simulink model "test4"  (R2021a)
settings: Solver=VariableStepAuto  StartTime=0.0  StopTime=20  RelTol=1e-1
undefined symbols (not defined in the file): B_EMB, C1, C_EMB, D_EMB, f, i_EMB, JL, JM, Jm_EMB, K1, N_EMB, rb_EMB, s_EMB, sigbuilder_block, Tc_EMB, Ts_EMB, ub_EMB
libraries: powerlib_extras x9, spsDCVoltageSourceLib x5, spsPermanentMagnetSynchronousMachineLib x5, spsUniversalBridgeLib x5, spspowerguiLib x5, spsVoltageMeasurementLib x4, pid_lib x4, simulink x3, dsparch4 x2, instrumentlib x2, Solver_SF x1
(part 1 of 3)
settings Model: Creator=86188  LastModifiedBy=86188
settings DataIOCC: ReturnWorkspaceOutputs=off

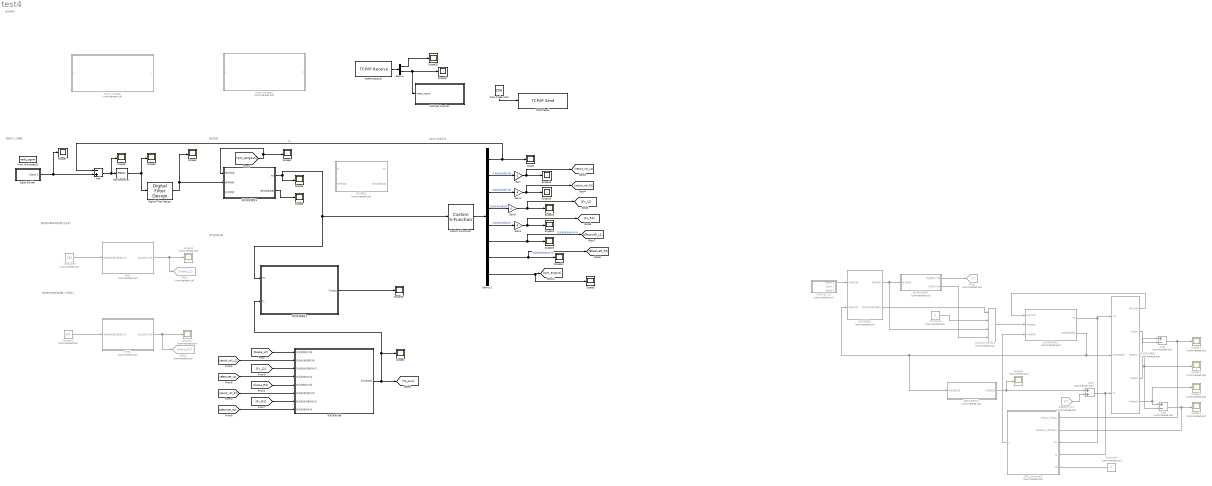
== system test4 ==
  note: 传动系统仿真
  note: 驱动电机
  note: Carsim仿真平台
  note: 驾驶员/工况模型
  note: 线控制动EMB制动器(左后轮)
  note: 线控制动EMB制动器（右后轮）
  note: 驱动电机
  Add : Sum  Inputs=-+
  Add5 : Sum  Commented=on  Inputs=+-
  Add6 : Sum  Commented=on  Inputs=+-
  Add7 : Sum  Commented=on
  CarSim S-Function : Solver_SF/CarSim S-Function  Priority=1  SIMFILE=simfile.sim
  Constant2 : Constant  Commented=on  Value=600
  Constant3 : Constant  Commented=on  Value=0
  Constant4 : Constant  Commented=on  Value=0
  Constant5 : Constant  Commented=on  Value=600
  Demux : Demux  Outputs=2
  Demux1 : Demux  Outputs=8
  Digital Filter Design : dsparch4/Digital Filter Design  mwdsp_browser_bugfix_var=off
  EMB : Subsystem  Commented=on
  EMB1 : Subsystem  Commented=on
  From Workspace1 : FromWorkspace  VariableName=nedc_signal  SampleTime=-1
  Gain{,1,3..4} (4 alike) : Gain  Gain=-1
  Goto : Goto  Commented=on  GotoTag=brake_L2
  Goto1 : Goto  Commented=on  GotoTag=T
  Goto2 : Goto  Commented=on  GotoTag=brake_R2
  MATLAB Function : MATLAB Function  TreatAsAtomicUnit=on
  MPC_controller1 : MATLAB Function  Commented=on  TreatAsAtomicUnit=on
  Multiport Switch1 : MultiPortSwitch  Commented=on  DataPortOrder=Zero-based contiguous  zeroidx=on
  PID Controller : pid_lib/PID Controller  Controller=PID  Form=Parallel  TimeDomain=Continuous-time  UseExternalTs=off  SampleTime=-1  IntegratorMethod=Forward Euler  FilterMethod=Forward Euler  ControllerParametersSource=internal  P=200  I=100  D=0  UseFilter=on  N=100  TunerSelectOption=Transfer Function Based (PID Tuner App)  InitialConditionSource=internal  InitialConditionForIntegrator=0  InitialConditionForFilter=0  DifferentiatorICPrevScaledInput=0  ExternalReset=none  TrackingMode=off  Kt=1  LimitOutput=off  SatLimitsSource=internal  UpperSaturationLimit=3000  LowerSaturationLimit=-3000  LinearizeAsGain=on  AntiWindupMode=none  Kb=1  POutMin=[]  POutMax=[]  IOutMin=[]  IOutMax=[]  DOutMin=[]  DOutMax=[]  NOutMin=[]  NOutMax=[]  SumOutMin=[]  SumOutMax=[]  SaturationOutMin=[]  SaturationOutMax=[]  PParamMin=[]  PParamMax=[]  IParamMin=[]  IParamMax=[]  DParamMin=[]  DParamMax=[]  NParamMin=[]  NParamMax=[]  KbParamMin=[]  KbParamMax=[]  KtParamMin=[]  KtParamMax=[]  KbOutMin=[]  KbOutMax=[]  KtOutMin=[]  KtOutMax=[]  IntegratorOutMin=[]  IntegratorOutMax=[]  FilterOutMin=[]  FilterOutMax=[]  SumI1OutMin=[]  SumI1OutMax=[]  SumI2OutMin=[]  SumI2OutMax=[]  SumI3OutMin=[]  SumI3OutMax=[]  SumI4OutMin=[]  SumI4OutMax=[]  SumDOutMin=[]  SumDOutMax=[]  DifferentiatorOutMin=[]  DifferentiatorOutMax=[]  FilterDiffOutCoefMin=[]  FilterDiffOutCoefMax=[]  ReciprocalOutMin=[]  ReciprocalOutMax=[]  SumDenOutMin=[]  SumDenOutMax=[]  SumNumOutMin=[]  SumNumOutMax=[]  DivideOutMin=[]  DivideOutMax=[]  UdiffTsProdOutMin=[]  UdiffTsProdOutMax=[]  NTsProdOutMin=[]  NTsProdOutMax=[]  UintegralTsProdOutMin=[]  UintegralTsProdOutMax=[]  UngainTsProdOutMin=[]  UngainTsProdOutMax=[]  IntegratorContinuousStateAttributes=''  IntegratorStateMustResolveToSignalObject=off  IntegratorRTWStateStorageClass=Auto  FilterContinuousStateAttributes=''  FilterStateMustResolveToSignalObject=off  FilterRTWStateStorageClass=Auto  ParallelPVariant=InternalParameters  IdealPVariant=Disabled  IVariant=InternalParameters  DVariant=InternalParameters  IntegratorVariant=Continuous  SatVariant=Disabled  AWVariant=Passthrough  PCopyVariant=Disabled  TRVariant=Disabled  FdbkBlocksVariant=Forward  IdealPFdbkVariant=Disabled  SatFdbkVariant=Disabled  DerivativeFilterVariant=ContFilter  NVariant=InternalParameters  NCopyVariant=Disabled  FilterICVariant=InternalICsFilter  IntegratorICVariant=InternalICs  ExternalResetVariant=Disabled  TRSumVariant=Passthrough  SumFdbkVariant=Disabled  SumVariant=Sum_PID  TsampFilterVariant=InternalTs  TsampNgainVariant=Passthrough  TsampIntegralVariant=Passthrough  ExternalSaturationOutDataTypeStr=Inherit: Same as second input
  Scope{,1..9,16..19,21..25} (19 alike) : Scope
  Scope{10..15,20} (7 alike) : Scope  Commented=on
  Signal Builder : Subsystem  Tag=STV Subsys  LoadFcn=sigbuilder_block('load');  StartFcn=sigbuilder_block('start');  StopFcn=sigbuilder_block('stop');  ClipboardFcn=sigbuilder_block('clipboard');  mask(Sigbuilder block){tuvar=[0:10]}
      mask help: Simulink:masks:SigbuilderBlock_MD
      mask init:
      | if ~strcmp(get_param(bdroot(gcbh),'SimulationStatus'),'stopped') tuvar = sigbuilder_block('maskInit'); end
      settings: CopyFcn=sigbuilder_block('copy');  DeleteFcn=sigbuilder_block('delete');  ModelCloseFcn=sigbuilder_block('modelClose');  PreSaveFcn=sigbuilder_block('preSave');  PauseFcn=sigbuilder_block('pause');  ContinueFcn=sigbuilder_block('continue');  NameChangeFcn=sigbuilder_block('namechange');  OpenFcn=sigbuilder_block('open',[86.4 109.2 550.8 400.2 ]);  CloseFcn=sigbuilder_block('close');
      mask Display: plot(0, 0, 100, 100,[2, 2, 32, 32, 2], [68, 8, 8, 68, 68],[32, 2], [38, 38], [32, 19, 2],[53, 60, 44], [32, 17, 17, 2],[16, 16, 31, 31]);txt = getActiveGroup(gcbh);text(2, 100, txt,'verticalAlignment', 'top');
  TCP/IP Receive : instrumentlib/TCP//IP Receive  Host=127.0.0.1  Port=50001  DataSize="[1  2]"  EnableBlockingMode=on  Timeout=10  SampleTime=0.01  DataType=double  ByteOrder=LittleEndian  ASCIIFormatting=%f,  Terminator=LF
  TCP/IP Send : instrumentlib/TCP//IP Send  Host=127.0.0.1  Port=50000  EnableBlockingMode=on  Timeout=10  ByteOrder=LittleEndian  TransferDelay=on
  Zero-Order Hold : ZeroOrderHold  SampleTime=0.01
  brake_strategy : MATLAB Function  Commented=on  TreatAsAtomicUnit=on
  brake_strategy1 : MATLAB Function  Commented=on  TreatAsAtomicUnit=on
  传动系统模型1 : Subsystem
  传动系统模型2 : Subsystem  Commented=on
  复合制动策略1 : Subsystem  Commented=on
  机械制动力矩1 : From  Commented=on  GotoTag=T
  电机模型1 : Subsystem  Commented=on
  行驶车速工况1 : Subsystem  Tag=STV Subsys  Commented=on  LoadFcn=sigbuilder_block('load');  StartFcn=sigbuilder_block('start');  StopFcn=sigbuilder_block('stop');  ClipboardFcn=sigbuilder_block('clipboard');  mask(Sigbuilder block){tuvar=[0:10]}
      mask help: Simulink:masks:SigbuilderBlock_MD
      mask init:
      | if ~strcmp(get_param(bdroot(gcbh),'SimulationStatus'),'stopped') tuvar = sigbuilder_block('maskInit'); end
      settings: CopyFcn=sigbuilder_block('copy');  DeleteFcn=sigbuilder_block('delete');  ModelCloseFcn=sigbuilder_block('modelClose');  PreSaveFcn=sigbuilder_block('preSave');  PauseFcn=sigbuilder_block('pause');  ContinueFcn=sigbuilder_block('continue');  NameChangeFcn=sigbuilder_block('namechange');  OpenFcn=sigbuilder_block('open',[5.4 36 1141.2 517.8 ]);  CloseFcn=sigbuilder_block('close');
      mask Display: plot(0, 0, 100, 100,[2, 2, 32, 32, 2], [68, 8, 8, 68, 68],[32, 2], [38, 38], [32, 19, 2],[53, 60, 44], [32, 17, 17, 2],[16, 16, 31, 31]);txt = getActiveGroup(gcbh);text(2, 100, txt,'verticalAlignment', 'top');
  路面负载转矩1 : Subsystem  Commented=on
  车轮负载计算 : Subsystem
  驱动电机模型1 : Subsystem  Commented=on
  驱动电机模型4 : Subsystem
  驾驶员模型1 : Subsystem  Commented=on
  wires:
  CarSim S-Function/1 -> Demux1/1
  MPC_controller1/1(u) -> 驱动电机模型1/3(补偿转矩)
  传动系统模型2/3(dthetaL) -> Add5/2, Scope11/1
  Add6/1 -> MPC_controller1/1(thetaM_thetaL), Scope13/1
  传动系统模型2/2(thetaL) -> Add6/2
  传动系统模型2/4(thetaM) -> Add6/1
  Multiport Switch1/1 -> 驱动电机模型1/2(参考转矩)
  驱动电机模型1/1(Te) -> 传动系统模型2/1(TM), MPC_controller1/3(TM)
  行驶车速工况1/1(Signal 1) -> 驾驶员模型1/1(参考转速)
  路面负载转矩1/1(负载转矩) -> Scope10/1, Add7/1
  驱动电机模型1/2(电机轴角速度) -> 传动系统模型2/2(电机轴转速), 驾驶员模型1/2(电机转速), 路面负载转矩1/1(电机轴转速)
  传动系统模型2/1(电机负载) -> 驱动电机模型1/1(电机负载)
  复合制动策略1/1(机械制动力矩) -> Goto1/1
  Constant4/1 -> MPC_controller1/5(ref)
  驾驶员模型1/1(参考转矩) -> 复合制动策略1/1(参考转矩), Multiport Switch1/3
  Add7/1 -> MPC_controller1/4(TL), 传动系统模型2/3(TL)
  复合制动策略1/2(电制动力矩) -> Multiport Switch1/4
  机械制动力矩1/1 -> Add7/2
  Constant3/1 -> Multiport Switch1/2
  传动系统模型2/5(dthetaM) -> Scope12/1, Add5/1
  Add5/1 -> MPC_controller1/2(dthetaM_dthetaLL), Scope14/1
  驾驶员模型1/2(电机驱动/制动模式) -> Multiport Switch1/1
  Demux1/1 -> Add/1, Scope/1  "Vx"
  Add/1 -> PID Controller/1, Scope2/1
  Signal Builder/1(Signal 1) -> Scope7/1, Add/2
  Demux1/3 -> Gain1/1  "右后轮滚动阻力矩"
  Demux1/2 -> Gain/1  "左后轮滚动阻力矩"
  Constant5/1 -> EMB/1(参考制动器分配制动力)
  EMB/1(输出制动力矩) -> Goto/1, Scope20/1
  Demux1/5 -> Gain4/1  "右后轮纵向驱动力"
  Demux1/4 -> Gain3/1  "左后轮纵向驱动力"
  EMB1/1(输出制动力矩) -> Goto2/1, Scope15/1
  Constant2/1 -> EMB1/1(参考制动器分配制动力)
  Demux1/6 -> [EfectiveR_L2], Scope23/1  "左后轮有效滚动半径"
  Demux1/7 -> [EfectiveR_R2], Scope24/1  "右后轮有效滚动半径"
  车轮负载计算/1(总负载转矩) -> Scope1/1, 传动系统模型1/2(TL), [TL_sum]
  [brake_R2] -> 车轮负载计算/5(右后轮制动力矩)
  [brake_L2] -> 车轮负载计算/1(左后轮制动力矩)
  [resisit_roll_L2] -> 车轮负载计算/2(左后轮滚动阻力矩)
  [resisit_roll_R2] -> 车轮负载计算/6(右后轮滚动阻力矩)
  [Fx_L2] -> 车轮负载计算/3(左后轮纵向驱动反力)
  [EfectiveR_L2] -> 车轮负载计算/4(左后轮有效半径)
  [Fx_R2] -> 车轮负载计算/7(右后轮纵向驱动反力)
  [EfectiveR_R2] -> 车轮负载计算/8(右后轮有效半径)
  Gain/1 -> Scope18/1, [resisit_roll_L2]
  Gain1/1 -> Scope19/1, [resisit_roll_R2]
  Gain3/1 -> [Fx_L2], Scope21/1
  Gain4/1 -> Scope22/1, [Fx_R2]
  PID Controller/1 -> Digital Filter Design/1, Scope3/1
  Demux1/8 -> [rpm_engout], Scope5/1
  Digital Filter Design/1 -> 驱动电机模型4/2(参考转矩), Scope4/1
  [rpm_engout] -> 驱动电机模型4/1(电机转速), Scope6/1
  驱动电机模型4/1(Te) -> Scope9/1, 传动系统模型1/1(TM), CarSim S-Function/1
  驱动电机模型4/2(电机轴角速度) -> Scope8/1
  传动系统模型1/1(Output) -> Scope16/1
  Demux/1 -> Scope25/1
  Demux/2 -> MATLAB Function/1(reset_signal), Scope17/1
  Zero-Order Hold/1 -> TCP/IP Send/1
  TCP/IP Receive/1 -> Demux/1

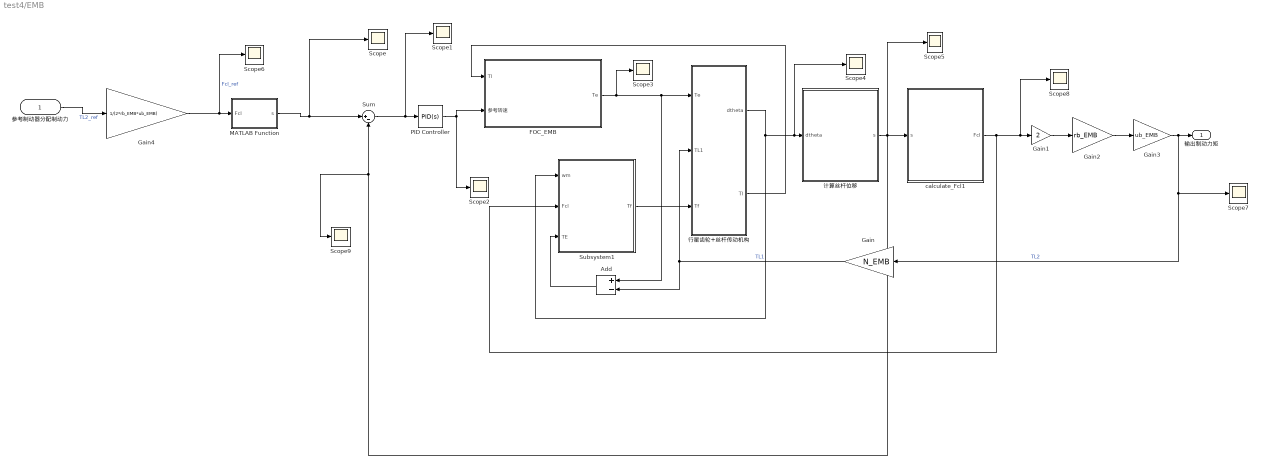
== system test4/EMB ==
  参考制动器分配制动力 : Inport
  Add : Sum  Inputs=+-
  FOC_EMB : Subsystem
  Gain : Gain  Gain=N_EMB
  Gain1 : Gain  Gain=2
  Gain2 : Gain  Gain=rb_EMB
  Gain3 : Gain  Gain=ub_EMB
  Gain4 : Gain  Gain=1/(2*rb_EMB*ub_EMB)
  MATLAB Function : MATLAB Function  TreatAsAtomicUnit=on
  PID Controller : pid_lib/PID Controller  Controller=PID  Form=Parallel  TimeDomain=Continuous-time  UseExternalTs=off  SampleTime=-1  IntegratorMethod=Forward Euler  FilterMethod=Forward Euler  ControllerParametersSource=internal  P=13000  I=150000  D=20  UseFilter=on  N=100  TunerSelectOption=Transfer Function Based (PID Tuner App)  InitialConditionSource=internal  InitialConditionForIntegrator=0  InitialConditionForFilter=0  DifferentiatorICPrevScaledInput=0  ExternalReset=none  TrackingMode=off  Kt=1  LimitOutput=off  SatLimitsSource=internal  UpperSaturationLimit=inf  LowerSaturationLimit=-inf  LinearizeAsGain=on  AntiWindupMode=none  Kb=1  POutMin=[]  POutMax=[]  IOutMin=[]  IOutMax=[]  DOutMin=[]  DOutMax=[]  NOutMin=[]  NOutMax=[]  SumOutMin=[]  SumOutMax=[]  SaturationOutMin=[]  SaturationOutMax=[]  PParamMin=[]  PParamMax=[]  IParamMin=[]  IParamMax=[]  DParamMin=[]  DParamMax=[]  NParamMin=[]  NParamMax=[]  KbParamMin=[]  KbParamMax=[]  KtParamMin=[]  KtParamMax=[]  KbOutMin=[]  KbOutMax=[]  KtOutMin=[]  KtOutMax=[]  IntegratorOutMin=[]  IntegratorOutMax=[]  FilterOutMin=[]  FilterOutMax=[]  SumI1OutMin=[]  SumI1OutMax=[]  SumI2OutMin=[]  SumI2OutMax=[]  SumI3OutMin=[]  SumI3OutMax=[]  SumI4OutMin=[]  SumI4OutMax=[]  SumDOutMin=[]  SumDOutMax=[]  DifferentiatorOutMin=[]  DifferentiatorOutMax=[]  FilterDiffOutCoefMin=[]  FilterDiffOutCoefMax=[]  ReciprocalOutMin=[]  ReciprocalOutMax=[]  SumDenOutMin=[]  SumDenOutMax=[]  SumNumOutMin=[]  SumNumOutMax=[]  DivideOutMin=[]  DivideOutMax=[]  UdiffTsProdOutMin=[]  UdiffTsProdOutMax=[]  NTsProdOutMin=[]  NTsProdOutMax=[]  UintegralTsProdOutMin=[]  UintegralTsProdOutMax=[]  UngainTsProdOutMin=[]  UngainTsProdOutMax=[]  IntegratorContinuousStateAttributes=''  IntegratorStateMustResolveToSignalObject=off  IntegratorRTWStateStorageClass=Auto  FilterContinuousStateAttributes=''  FilterStateMustResolveToSignalObject=off  FilterRTWStateStorageClass=Auto  ParallelPVariant=InternalParameters  IdealPVariant=Disabled  IVariant=InternalParameters  DVariant=InternalParameters  IntegratorVariant=Continuous  SatVariant=Disabled  AWVariant=Passthrough  PCopyVariant=Disabled  TRVariant=Disabled  FdbkBlocksVariant=Forward  IdealPFdbkVariant=Disabled  SatFdbkVariant=Disabled  DerivativeFilterVariant=ContFilter  NVariant=InternalParameters  NCopyVariant=Disabled  FilterICVariant=InternalICsFilter  IntegratorICVariant=InternalICs  ExternalResetVariant=Disabled  TRSumVariant=Passthrough  SumFdbkVariant=Disabled  SumVariant=Sum_PID  TsampFilterVariant=InternalTs  TsampNgainVariant=Passthrough  TsampIntegralVariant=Passthrough  ExternalSaturationOutDataTypeStr=Inherit: Same as second input
  Scope{,1..9} (10 alike) : Scope
  Subsystem1 : Subsystem
  Sum : Sum  Inputs=|+-
  calculate_Fcl1 : Subsystem
  行星齿轮+丝杆传动机构 : Subsystem
  计算丝杆位移 : Subsystem
  输出制动力矩 : Outport
  wires:
  FOC_EMB/1(Te) -> Add/1, 行星齿轮+丝杆传动机构/1(Te), Scope3/1
  Gain3/1 -> Gain/1, Scope7/1, 输出制动力矩/1  "TL2"
  Gain/1 -> Add/2, 行星齿轮+丝杆传动机构/2(TL1)  "TL1"
  Subsystem1/1(Tf) -> 行星齿轮+丝杆传动机构/3(Tf)
  行星齿轮+丝杆传动机构/1(dtheta) -> Subsystem1/1(wm), Scope4/1, 计算丝杆位移/1(dtheta)
  计算丝杆位移/1(s) -> calculate_Fcl1/1(s), Sum/2, Scope9/1, Scope5/1
  calculate_Fcl1/1(Fcl) -> Scope8/1, Gain1/1, Subsystem1/2(Fcl)
  Gain1/1 -> Gain2/1
  Gain2/1 -> Gain3/1
  Add/1 -> Subsystem1/3(TE)
  行星齿轮+丝杆传动机构/2(Tl) -> FOC_EMB/1(Tl)
  参考制动器分配制动力/1 -> Gain4/1  "TL2_ref"
  Sum/1 -> Scope1/1, PID Controller/1
  PID Controller/1 -> FOC_EMB/2(参考转速), Scope2/1
  MATLAB Function/1(s) -> Scope/1, Sum/1
  Gain4/1 -> Scope6/1, MATLAB Function/1(Fcl)  "Fcl_ref"

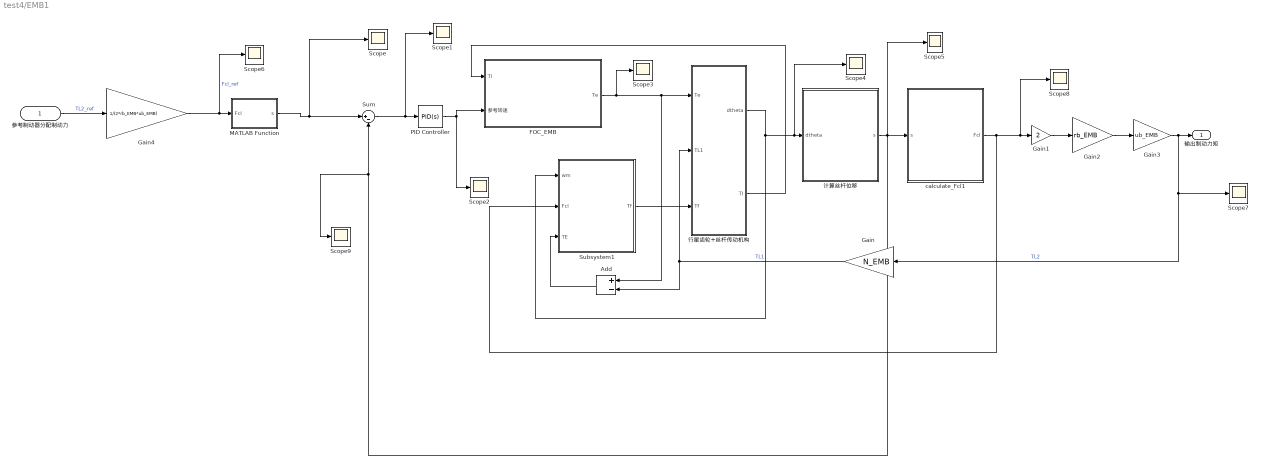
== system test4/EMB1 ==
  参考制动器分配制动力 : Inport
  Add : Sum  Inputs=+-
  FOC_EMB : Subsystem
  Gain : Gain  Gain=N_EMB
  Gain1 : Gain  Gain=2
  Gain2 : Gain  Gain=rb_EMB
  Gain3 : Gain  Gain=ub_EMB
  Gain4 : Gain  Gain=1/(2*rb_EMB*ub_EMB)
  MATLAB Function : MATLAB Function  TreatAsAtomicUnit=on
  PID Controller : pid_lib/PID Controller  Controller=PID  Form=Parallel  TimeDomain=Continuous-time  UseExternalTs=off  SampleTime=-1  IntegratorMethod=Forward Euler  FilterMethod=Forward Euler  ControllerParametersSource=internal  P=13000  I=150000  D=20  UseFilter=on  N=100  TunerSelectOption=Transfer Function Based (PID Tuner App)  InitialConditionSource=internal  InitialConditionForIntegrator=0  InitialConditionForFilter=0  DifferentiatorICPrevScaledInput=0  ExternalReset=none  TrackingMode=off  Kt=1  LimitOutput=off  SatLimitsSource=internal  UpperSaturationLimit=inf  LowerSaturationLimit=-inf  LinearizeAsGain=on  AntiWindupMode=none  Kb=1  POutMin=[]  POutMax=[]  IOutMin=[]  IOutMax=[]  DOutMin=[]  DOutMax=[]  NOutMin=[]  NOutMax=[]  SumOutMin=[]  SumOutMax=[]  SaturationOutMin=[]  SaturationOutMax=[]  PParamMin=[]  PParamMax=[]  IParamMin=[]  IParamMax=[]  DParamMin=[]  DParamMax=[]  NParamMin=[]  NParamMax=[]  KbParamMin=[]  KbParamMax=[]  KtParamMin=[]  KtParamMax=[]  KbOutMin=[]  KbOutMax=[]  KtOutMin=[]  KtOutMax=[]  IntegratorOutMin=[]  IntegratorOutMax=[]  FilterOutMin=[]  FilterOutMax=[]  SumI1OutMin=[]  SumI1OutMax=[]  SumI2OutMin=[]  SumI2OutMax=[]  SumI3OutMin=[]  SumI3OutMax=[]  SumI4OutMin=[]  SumI4OutMax=[]  SumDOutMin=[]  SumDOutMax=[]  DifferentiatorOutMin=[]  DifferentiatorOutMax=[]  FilterDiffOutCoefMin=[]  FilterDiffOutCoefMax=[]  ReciprocalOutMin=[]  ReciprocalOutMax=[]  SumDenOutMin=[]  SumDenOutMax=[]  SumNumOutMin=[]  SumNumOutMax=[]  DivideOutMin=[]  DivideOutMax=[]  UdiffTsProdOutMin=[]  UdiffTsProdOutMax=[]  NTsProdOutMin=[]  NTsProdOutMax=[]  UintegralTsProdOutMin=[]  UintegralTsProdOutMax=[]  UngainTsProdOutMin=[]  UngainTsProdOutMax=[]  IntegratorContinuousStateAttributes=''  IntegratorStateMustResolveToSignalObject=off  IntegratorRTWStateStorageClass=Auto  FilterContinuousStateAttributes=''  FilterStateMustResolveToSignalObject=off  FilterRTWStateStorageClass=Auto  ParallelPVariant=InternalParameters  IdealPVariant=Disabled  IVariant=InternalParameters  DVariant=InternalParameters  IntegratorVariant=Continuous  SatVariant=Disabled  AWVariant=Passthrough  PCopyVariant=Disabled  TRVariant=Disabled  FdbkBlocksVariant=Forward  IdealPFdbkVariant=Disabled  SatFdbkVariant=Disabled  DerivativeFilterVariant=ContFilter  NVariant=InternalParameters  NCopyVariant=Disabled  FilterICVariant=InternalICsFilter  IntegratorICVariant=InternalICs  ExternalResetVariant=Disabled  TRSumVariant=Passthrough  SumFdbkVariant=Disabled  SumVariant=Sum_PID  TsampFilterVariant=InternalTs  TsampNgainVariant=Passthrough  TsampIntegralVariant=Passthrough  ExternalSaturationOutDataTypeStr=Inherit: Same as second input
  Scope{,1..9} (10 alike) : Scope
  Subsystem1 : Subsystem
  Sum : Sum  Inputs=|+-
  calculate_Fcl1 : Subsystem
  行星齿轮+丝杆传动机构 : Subsystem
  计算丝杆位移 : Subsystem
  输出制动力矩 : Outport
  wires:
  Gain4/1 -> MATLAB Function/1(Fcl), Scope6/1  "Fcl_ref"
  MATLAB Function/1(s) -> Sum/1, Scope/1
  PID Controller/1 -> Scope2/1, FOC_EMB/2(参考转速)
  Sum/1 -> PID Controller/1, Scope1/1
  参考制动器分配制动力/1 -> Gain4/1  "TL2_ref"
  行星齿轮+丝杆传动机构/2(Tl) -> FOC_EMB/1(Tl)
  Add/1 -> Subsystem1/3(TE)
  Gain2/1 -> Gain3/1
  Gain1/1 -> Gain2/1
  calculate_Fcl1/1(Fcl) -> Subsystem1/2(Fcl), Gain1/1, Scope8/1
  计算丝杆位移/1(s) -> Scope5/1, Scope9/1, Sum/2, calculate_Fcl1/1(s)
  行星齿轮+丝杆传动机构/1(dtheta) -> 计算丝杆位移/1(dtheta), Scope4/1, Subsystem1/1(wm)
  Subsystem1/1(Tf) -> 行星齿轮+丝杆传动机构/3(Tf)
  Gain/1 -> 行星齿轮+丝杆传动机构/2(TL1), Add/2  "TL1"
  Gain3/1 -> 输出制动力矩/1, Scope7/1, Gain/1  "TL2"
  FOC_EMB/1(Te) -> Scope3/1, 行星齿轮+丝杆传动机构/1(Te), Add/1

== system test4/Signal Builder ==
  Demux : Demux  Tag=STV Demux  Outputs=1
      settings: DisplayOption=none
  FromWs : FromWorkspace  Tag=STV FromWs  VariableName=tuvar
      SigBuilderData=|
      | common.afterFinalStr = 'Extrapolate'
      | common.sampleTime = 0
      | dataSet.timeRange = [0 10]
      | dataSet.name = 'Group 1'
      | sbobj.Groups.Name = 'Group 1'
      | sbobj.Groups.Signals.Name = 'Signal 1'
      | sbobj.Groups.Signals.XData = [0 4 6 8 10]
      | sbobj.Groups.Signals.YData = [0 40 40 0 0]
  Signal 1 : Outport  Tag=STV Outport
  wires:
  Demux/1 -> Signal 1/1
  FromWs/1 -> Demux/1

== system test4/传动系统模型1 ==
  TM : Inport
  TL : Inport  Port=2
  Add : Sum  Inputs=+-
  Fcn1 : Subsystem
  Fcn2 : Subsystem
  Output : Outport
  wires:
  Fcn2/1(d2thetaL) -> Fcn1/2(d2theta1)
  TM/1 -> Fcn1/1(TM)
  Fcn1/1(d2theta) -> Fcn2/2(d2thata)
  TL/1 -> Fcn2/1(TL)
  Add/1 -> Output/1
  Fcn2/2(dthetaL) -> Add/1
  Fcn1/2(dtheta) -> Add/2

== system test4/传动系统模型2 ==
  TM : Inport
  电机轴转速 : Inport  Port=2
  TL : Inport  Port=3
  Fcn1 : Subsystem
  Fcn2 : Subsystem
  轮胎模型 : Subsystem
  电机负载 : Outport
  thetaL : Outport  Port=2
  dthetaL : Outport  Port=3
  thetaM : Outport  Port=4
  dthetaM : Outport  Port=5
  wires:
  Fcn2/3(dthetaL) -> 轮胎模型/1(Input), dthetaL/1
  Fcn2/2(thetaL) -> thetaL/1
  TL/1 -> Fcn2/1(TL)
  Fcn1/4(dthetaM) -> dthetaM/1
  Fcn1/3(thetaM) -> thetaM/1
  Fcn1/2(电机负载) -> 电机负载/1
  Fcn1/1(d2theta) -> Fcn2/2(d2thata)
  电机轴转速/1 -> Fcn1/3(电机轴转速)
  TM/1 -> Fcn1/1(TM)
  Fcn2/1(d2thetaL) -> Fcn1/2(d2theta1)

== system test4/复合制动策略1 ==
  参考转矩 : Inport
  Constant : Constant  Value=0
  Switch : Switch
  机械制动力矩 : Outport
  电制动力矩 : Outport  Port=2
  wires:
  Switch/1 -> 电制动力矩/1
  Constant/1 -> Switch/1
  参考转矩/1 -> Switch/2, Switch/3

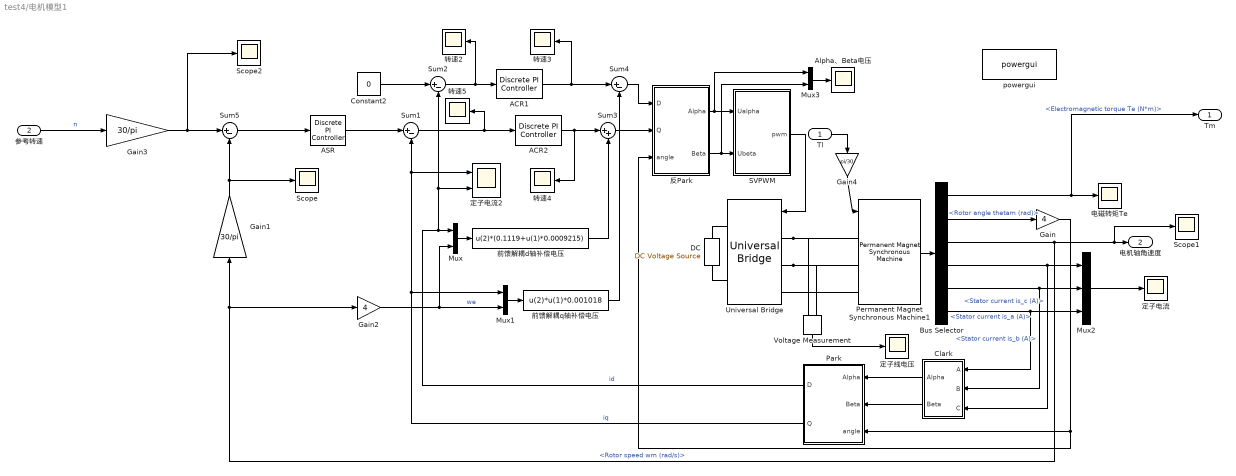
== system test4/电机模型1 ==
  Tl : Inport
  参考转速 : Inport  Port=2
  ACR1 : powerlib_extras/Discrete  Control Blocks/Discrete PI Controller  Kp=4  Ki=80  Par_Limits=[760*0.9*sqrt(1/3) -760*0.9*sqrt(1/3)]  Init=0  Ts=1e-6
  ACR2 : powerlib_extras/Discrete  Control Blocks/Discrete PI Controller  Kp=4  Ki=80  Par_Limits=[760*0.9*sqrt(1/3) -760*0.9*sqrt(1/3)]  Init=0  Ts=1e-6
  ASR : powerlib_extras/Discrete  Control Blocks/Discrete PI Controller  Kp=5  Ki=200  Par_Limits=[1000 -1000]  Init=0  Ts=1e-6
  Alpha、Beta电压 : Scope
  Bus Selector : BusSelector  OutputSignals=Electromagnetic torque Te (N*m),Rotor angle thetam (rad),Rotor speed wm (rad/s),Stator current is_c (A),Stator current is_b (A),Stator current is_a (A)
  Clark : Subsystem
  Constant2 : Constant  Value=0
  DC : spsDCVoltageSourceLib/DC Voltage Source  Amplitude=560  Measurements=None
  Gain : Gain  Gain=4
  Gain1 : Gain  Gain=30/pi
  Gain2 : Gain  Gain=4
  Gain3 : Gain  Gain=30/pi
  Gain4 : Gain  Gain=pi/30
  Mux : Mux  Inputs=2
  Mux1 : Mux  Inputs=2
  Mux2 : Mux  Inputs=3
  Mux3 : Mux  Inputs=2
  Park : Subsystem
  Permanent Magnet Synchronous Machine1 : spsPermanentMagnetSynchronousMachineLib/Permanent Magnet Synchronous Machine  NbPhases=3  FluxDistribution=Sinusoidal  RotorType=Salient-pole  MechanicalLoad=Speed w  PresetModel=No  ShowDetailedParameters=on  MeasurementBus=off  Resistance=0.01  Inductance=8.5e-3  dqInductances=[0.0009215 0.001018]  La=0.000835  MachineConstant=Flux linkage established by magnets (V.s)  Flux=0.1  VoltageCst=72.552  TorqueCst=0.6  Flat=120  Mechanical=[0.04 0.0002024 4 0]  PolePairs=4  InitialConditions=[0,0, 0,0]  InitialConditions5ph=[0 0 0 0 0 0]  RefAngle=Aligned with phase A axis (original Park)  IterativeDiscreteModel=Trapezoidal non iterative  TsBlock=-1  TsPowergui=0
  SVPWM : Subsystem
  Scope : Scope
  Scope1 : Scope
  Scope2 : Scope
  Sum{1..2,4..5} (4 alike) : Sum  Inputs=|+-
  Sum3 : Sum  Inputs=|++
  Universal Bridge : spsUniversalBridgeLib/Universal Bridge  Arms=3  SnubberResistance=1e5  SnubberCapacitance=inf  Device=IGBT / Diodes  Ron=1e-3  Lon=0  ForwardVoltages="[  0  0  ]"  ForwardVoltage=0  GTOparameters=[ 10e-6 , 20e-6 ]  IGBTparameters=[ 1e-6 , 2e-6 ]  Measurements=None  Measurements_2=None  converterType=Rectifier
  Voltage Measurement : spsVoltageMeasurementLib/Voltage Measurement  PhasorSimulation=off  OutputType=Complex  PSBequivalent=0
  powergui : spspowerguiLib/powergui  Priority=1  SimulationMode=Discrete  SampleTime=1e-6  frequency=60  Iterations=50  frequencyindice=0  Pbase=100e6  ErrMax=1e-4  UnitsV=kV  UnitsW=MW  buscounter=0  FunctionMessages=off  echomessages=off  EnableUseOfTLC=off  CurrentSourceSwitches=off  DisableSnubberDevices=off  DisableRonSwitches=off  DisableVfSwitches=off  DisplayEquations=off  AutomaticDiscreteSolvers=off  SolverType=Tustin  Interpol=off  ExternalGateDelay=off  methode=off  Ts=0  x0status=blocks  SPID=off  SwTol=0  HookPort=off  NonlinearTolerance=1e-4  nMaxIteration=100  ContinueOnMaxIteration=off  RestoreLinks=warning  ResistiveCurrentMeasurement=off  Frange=[0:2:500]  Ylog=off  Xlog=on  ShowGrid=off  save=off  variable=ZData  structure=ScopeData7  ZoomFFT=on  StartTime=2.5  cycles=3  DisplayStyle=1  fundamental=60  FreqAxis=off  MaxFrequency=2000  frequencyindicesteady=1  RmsSteady=1  display=off
  前馈解耦d轴补偿电压 : Fcn  Expr=u(2)*(0.1119+u(1)*0.0009215)
  前馈解耦q轴补偿电压 : Fcn  Expr=u(2)*u(1)*0.001018
  反Park : Subsystem
  定子电流 : Scope
  定子电流2 : Scope  NumInputPorts=2
  定子线电压 : Scope
  电磁转矩Te : Scope
  转速{2..5} (4 alike) : Scope
  Tm : Outport
  电机轴角速度 : Outport  Port=2
  wires:
  Gain4/1 -> Permanent Magnet Synchronous Machine1/1
  ACR1/1 -> 转速3/1, Sum4/1
  Bus Selector/4 -> Mux2/1, Clark/3(C)  "<Stator current is_c (A)>"
  Constant2/1 -> Sum2/1
  Gain/1 -> 反Park/3(angle), Park/3(angle)
  Gain2/1 -> Mux1/2, Mux/2  "we"
  Mux1/1 -> 前馈解耦q轴补偿电压/1
  SVPWM/1(pwm) -> Universal Bridge/1
  Sum4/1 -> 反Park/1(D)
  ACR2/1 -> 转速4/1, Sum3/1
  前馈解耦d轴补偿电压/1 -> Sum3/2
  参考转速/1 -> Gain3/1  "n"
  Bus Selector/2 -> Gain/1  "<Rotor angle thetam (rad)>"
  Bus Selector/5 -> Mux2/2, Clark/2(B)  "<Stator current is_b (A)>"
  Bus Selector/1 -> Tm/1, 电磁转矩Te/1  "<Electromagnetic torque Te (N*m)>"
  Park/1(D) -> 定子电流2/2, Sum2/2, Mux/1  "id"
  Sum3/1 -> 反Park/2(Q)
  反Park/2(Beta) -> Mux3/2, SVPWM/2(Ubeta)
  Mux/1 -> 前馈解耦d轴补偿电压/1
  Bus Selector/3 -> Gain2/1, Gain1/1, Scope1/1, 电机轴角速度/1  "<Rotor speed wm (rad/s)>"
  反Park/1(Alpha) -> Mux3/1, SVPWM/1(Ualpha)
  Mux3/1 -> Alpha、Beta电压/1
  Sum1/1 -> 转速5/1, ACR2/1
  Clark/2(Beta) -> Park/2(Beta)
  Park/2(Q) -> Mux1/1, 定子电流2/1, Sum1/2  "iq"
  Permanent Magnet Synchronous Machine1/1 -> Bus Selector/1
  Clark/1(Alpha) -> Park/1(Alpha)
  Sum5/1 -> ASR/1
  Bus Selector/6 -> Mux2/3, Clark/1(A)  "<Stator current is_a (A)>"
  Mux2/1 -> 定子电流/1
  Sum2/1 -> 转速2/1, ACR1/1
  前馈解耦q轴补偿电压/1 -> Sum4/2
  Voltage Measurement/1 -> 定子线电压/1
  Tl/1 -> Gain4/1
  ASR/1 -> Sum1/1
  Gain1/1 -> Sum5/2, Scope/1
  Gain3/1 -> Scope2/1, Sum5/1
  connections:
  DC/LConn1 -- Universal Bridge/RConn2
  Permanent Magnet Synchronous Machine1/LConn3 -- Universal Bridge/LConn3
  DC/RConn1 -- Universal Bridge/RConn1
  Universal Bridge/LConn2 -- Permanent Magnet Synchronous Machine1/LConn2 -- Voltage Measurement/LConn2
  Universal Bridge/LConn1 -- Permanent Magnet Synchronous Machine1/LConn1 -- Voltage Measurement/LConn1

== system test4/行驶车速工况1 ==
  Demux : Demux  Tag=STV Demux  Outputs=3
      settings: DisplayOption=none
  FromWs : FromWorkspace  Tag=STV FromWs  VariableName=tuvar
      SigBuilderData=|
      | common.afterFinalStr = 'Extrapolate'
      | common.sampleTime = 0
      | dataSet.timeRange = [0 10]
      | dataSet.name = 'Group 1'
      | sbobj.Groups.Name = 'Group 1'
      | sbobj.Groups.Signals(1).Name = 'Signal 1'
      | sbobj.Groups.Signals(1).XData = [0 2 3 10]
      | sbobj.Groups.Signals(1).YData = [1000 1000 0 0]
      | sbobj.Groups.Signals(2).Name = 'Signal 2'
      | sbobj.Groups.Signals(2).XData = [0 2 2 3 3 10]
      | sbobj.Groups.Signals(2).YData = [10 10 50 50 10 10]
      | sbobj.Groups.Signals(3).Name = 'Signal 3'
      | sbobj.Groups.Signals(3).XData = [0 10]
      | sbobj.Groups.Signals(3).YData = [10 10]
  Signal 1 : Outport  Tag=STV Outport
  Signal 2 : Outport  Tag=STV Outport  Port=2
  Signal 3 : Outport  Tag=STV Outport  Port=3
  wires:
  Demux/3 -> Signal 3/1
  Demux/2 -> Signal 2/1
  Demux/1 -> Signal 1/1
  FromWs/1 -> Demux/1

== system test4/路面负载转矩1 ==
  电机轴转速 : Inport
  Constant2 : Constant
  Constant3 : Constant  Value=0
  Product : Product
  Switch : Switch  Criteria=u2 > Threshold  Threshold=0.001
  负载 : Subsystem  Tag=STV Subsys  LoadFcn=sigbuilder_block('load');  StartFcn=sigbuilder_block('start');  StopFcn=sigbuilder_block('stop');  ClipboardFcn=sigbuilder_block('clipboard');  mask(Sigbuilder block){tuvar=[0:10]}
      mask help: Simulink:masks:SigbuilderBlock_MD
      mask init:
      | if ~strcmp(get_param(bdroot(gcbh),'SimulationStatus'),'stopped') tuvar = sigbuilder_block('maskInit'); end
      settings: CopyFcn=sigbuilder_block('copy');  DeleteFcn=sigbuilder_block('delete');  ModelCloseFcn=sigbuilder_block('modelClose');  PreSaveFcn=sigbuilder_block('preSave');  PauseFcn=sigbuilder_block('pause');  ContinueFcn=sigbuilder_block('continue');  NameChangeFcn=sigbuilder_block('namechange');  OpenFcn=sigbuilder_block('open',[5.4 36 1141.2 517.8 ]);  CloseFcn=sigbuilder_block('close');
      mask Display: plot(0, 0, 100, 100,[2, 2, 32, 32, 2], [68, 8, 8, 68, 68],[32, 2], [38, 38], [32, 19, 2],[53, 60, 44], [32, 17, 17, 2],[16, 16, 31, 31]);txt = getActiveGroup(gcbh);text(2, 100, txt,'verticalAlignment', 'top');
  负载转矩 : Outport
  wires:
  电机轴转速/1 -> Switch/2
  Constant2/1 -> Switch/1
  Product/1 -> 负载转矩/1
  负载/3(Signal 3) -> Product/1
  Constant3/1 -> Switch/3
  Switch/1 -> Product/2

== system test4/车轮负载计算 ==
  左后轮制动力矩 : Inport
  左后轮滚动阻力矩 : Inport  Port=2
  左后轮纵向驱动反力 : Inport  Port=3
  左后轮有效半径 : Inport  Port=4
  右后轮制动力矩 : Inport  Port=5
  右后轮滚动阻力矩 : Inport  Port=6
  右后轮纵向驱动反力 : Inport  Port=7
  右后轮有效半径 : Inport  Port=8
  Add : Sum  Inputs=+++
  Add1 : Sum  Inputs=+++
  Add2 : Sum
  Gain : Gain  Gain=0.001
  Gain1 : Gain  Gain=0.001
  Product1 : Product
  Product2 : Product
  Scope : Scope
  Scope1 : Scope
  总负载转矩 : Outport
  wires:
  左后轮纵向驱动反力/1 -> Product2/1
  左后轮有效半径/1 -> Gain1/1
  右后轮纵向驱动反力/1 -> Product1/1
  右后轮有效半径/1 -> Gain/1
  左后轮制动力矩/1 -> Add/1
  Product2/1 -> Add/3
  左后轮滚动阻力矩/1 -> Add/2
  右后轮制动力矩/1 -> Add1/1
  右后轮滚动阻力矩/1 -> Add1/2
  Product1/1 -> Add1/3
  Add/1 -> Add2/1, Scope/1
  Add1/1 -> Add2/2, Scope1/1
  Add2/1 -> 总负载转矩/1
  Gain/1 -> Product1/2
  Gain1/1 -> Product2/2

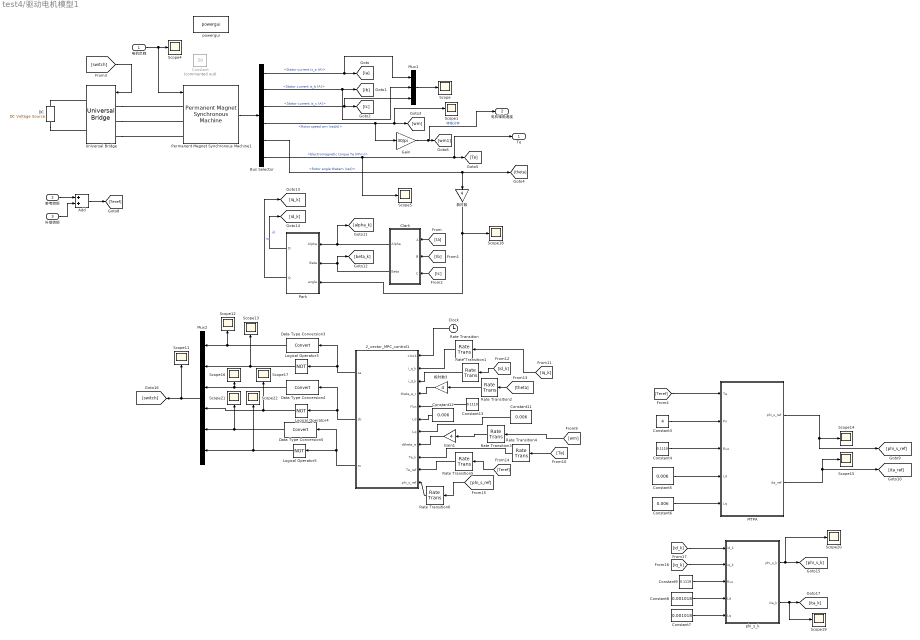
== system test4/驱动电机模型1 ==
  电机负载 : Inport
  参考转矩 : Inport  Port=2
  补偿转矩 : Inport  Port=3
  2_vector_MPC_control1 : MATLAB Function  TreatAsAtomicUnit=on  SystemSampleTime=1e-5
  Add : Sum
  Bus Selector : BusSelector  OutputSignals=Stator current is_a (A),Stator current is_b (A),Stator current is_c (A),Rotor speed wm (rad/s),Rotor angle thetam (rad),Electromagnetic torque Te (N*m)
  Clark : Subsystem
  Clock : Clock
  Constant : Constant  Commented=on  Value=50
  Constant{5..6,11..12} (4 alike) : Constant  Value=0.006
  Constant13 : Constant  Value=0.1119
  Constant3 : Constant  Value=4
  Constant4 : Constant  Value=0.1119
  Constant7 : Constant  Value=0.001018
  Constant8 : Constant  Value=0.001018
  Constant9 : Constant  Value=0.1119
  DC : spsDCVoltageSourceLib/DC Voltage Source  Amplitude=400  Measurements=None
  Data Type Conversion3 : DataTypeConversion
  Data Type Conversion4 : DataTypeConversion
  Data Type Conversion5 : DataTypeConversion
  Gain : Gain  Gain=30/pi
  Gain1 : Gain  Gain=4
  Logical Operator3 : Logic  Operator=NOT  AllPortsSameDT=off  OutDataTypeStr=boolean
  Logical Operator4 : Logic  Operator=NOT  AllPortsSameDT=off  OutDataTypeStr=boolean
  Logical Operator5 : Logic  Operator=NOT  AllPortsSameDT=off  OutDataTypeStr=boolean
  MTPA : MATLAB Function  TreatAsAtomicUnit=on
  Mux1 : Mux  Inputs=3
  Mux2 : Mux  Inputs=6
  Park : Subsystem
  Permanent Magnet Synchronous Machine1 : spsPermanentMagnetSynchronousMachineLib/Permanent Magnet Synchronous Machine  NbPhases=3  FluxDistribution=Sinusoidal  RotorType=Salient-pole  MechanicalLoad=Torque Tm  PresetModel=No  ShowDetailedParameters=on  MeasurementBus=off  Resistance=0.11  Inductance=8.5e-3  dqInductances=[0.006 0.006]  La=0.000835  MachineConstant=Flux linkage established by magnets (V.s)  Flux=0.1119  VoltageCst=81.1857  TorqueCst=0.6714  Flat=120  Mechanical=[0.04 0.0002024 4 0]  PolePairs=4  InitialConditions=[0,0, 0,0]  InitialConditions5ph=[0 0 0 0 0 0]  RefAngle=Aligned with phase A axis (original Park)  IterativeDiscreteModel=Trapezoidal non iterative  TsBlock=-1  TsPowergui=0
  Rate Transition : RateTransition  OutPortSampleTime=1e-5
  Rate Transition1 : RateTransition  OutPortSampleTime=1e-5
  Rate Transition2 : RateTransition  OutPortSampleTime=1e-5
  Rate Transition{3..6} (4 alike) : RateTransition  OutPortSampleTime=1e-4
  Scope{,1,4..5,11..22} (16 alike) : Scope
  Universal Bridge : spsUniversalBridgeLib/Universal Bridge  Arms=3  SnubberResistance=1e5  SnubberCapacitance=inf  Device=IGBT / Diodes  Ron=1e-3  Lon=0  ForwardVoltages="[  0  0  ]"  ForwardVoltage=0  GTOparameters=[ 10e-6 , 20e-6 ]  IGBTparameters=[ 1e-6 , 2e-6 ]  Measurements=None  Measurements_2=None  converterType=Rectifier
  phi_s_k : MATLAB Function  TreatAsAtomicUnit=on
  powergui : spspowerguiLib/powergui  Priority=1  SimulationMode=Discrete  SampleTime=1e-6  frequency=60  Iterations=50  frequencyindice=0  Pbase=100e6  ErrMax=1e-4  UnitsV=kV  UnitsW=MW  buscounter=0  FunctionMessages=off  echomessages=off  EnableUseOfTLC=off  CurrentSourceSwitches=off  DisableSnubberDevices=off  DisableRonSwitches=off  DisableVfSwitches=off  DisplayEquations=off  AutomaticDiscreteSolvers=off  SolverType=Tustin/Backward Euler (TBE)  Interpol=off  ExternalGateDelay=off  methode=off  Ts=100  x0status=blocks  SPID=on  SwTol=0  HookPort=off  NonlinearTolerance=1e-4  nMaxIteration=100  ContinueOnMaxIteration=off  RestoreLinks=warning  ResistiveCurrentMeasurement=off  Frange=[0:2:500]  Ylog=off  Xlog=on  ShowGrid=off  save=off  variable=ZData  structure=0  ZoomFFT=off  StartTime=0.0  cycles=1  DisplayStyle=1  fundamental=60  FreqAxis=off  MaxFrequency=1000  frequencyindicesteady=1  RmsSteady=1  display=off
  极对数 : Gain  Gain=4
  极对数3 : Gain  Gain=4
  Te : Outport
  电机轴角速度 : Outport  Port=2
  wires:
  电机负载/1 -> Scope4/1, Permanent Magnet Synchronous Machine1/1
  Rate Transition6/1 -> 2_vector_MPC_control1/11(phi_s_ref)
  Rate Transition5/1 -> 2_vector_MPC_control1/10(Te_ref)
  Rate Transition4/1 -> 2_vector_MPC_control1/9(Te_k)
  Rate Transition3/1 -> Gain1/1
  Rate Transition2/1 -> 极对数3/1
  Rate Transition1/1 -> 2_vector_MPC_control1/3(i_d_k)
  Rate Transition/1 -> 2_vector_MPC_control1/2(i_q_k)
  phi_s_k/2(ita_k) -> [ita_k], Scope19/1
  极对数3/1 -> 2_vector_MPC_control1/4(theta_e_r)
  Mux2/1 -> [switch], Scope11/1
  Logical Operator5/1 -> Scope22/1, Mux2/6
  Data Type Conversion5/1 -> Scope21/1, Mux2/5
  Logical Operator4/1 -> Scope17/1, Mux2/4
  Data Type Conversion4/1 -> Scope16/1, Mux2/3
  Logical Operator3/1 -> Scope13/1, Mux2/2
  Data Type Conversion3/1 -> Scope12/1, Mux2/1
  2_vector_MPC_control1/3(sc) -> Logical Operator5/1, Data Type Conversion5/1
  2_vector_MPC_control1/2(sb) -> Logical Operator4/1, Data Type Conversion4/1
  2_vector_MPC_control1/1(sa) -> Logical Operator3/1, Data Type Conversion3/1
  [id_k] -> phi_s_k/1(id_k)
  [iq_k] -> phi_s_k/2(iq_k)
  phi_s_k/1(phi_s_k) -> Scope20/1, [phi_s_k]
  Constant9/1 -> phi_s_k/3(flux)
  Constant8/1 -> phi_s_k/4(Ld)
  Constant7/1 -> phi_s_k/5(Lq)
  MTPA/1(phi_s_ref) -> Scope14/1, [phi_s_ref]
  MTPA/2(ita_ref) -> [ita_ref], Scope15/1
  Constant6/1 -> MTPA/5(Lq)
  Constant5/1 -> MTPA/4(Ld)
  Constant4/1 -> MTPA/3(flux)
  Constant3/1 -> MTPA/2(Pn)
  [Teref] -> MTPA/1(Te)
  Clock/1 -> 2_vector_MPC_control1/1(clock)
  Permanent Magnet Synchronous Machine1/1 -> Bus Selector/1
  Bus Selector/1 -> Mux1/1, [Ia]  "<Stator current is_a (A)>"
  Bus Selector/2 -> Mux1/2, [Ib]  "<Stator current is_b (A)>"
  Bus Selector/3 -> Mux1/3, [Ic]  "<Stator current is_c (A)>"
  Bus Selector/4 -> Gain/1, Scope1/1, [wm]  "<Rotor speed wm (rad/s)>"
  Bus Selector/5 -> 极对数/1, [theta]  "<Rotor angle thetam (rad)>"
  Bus Selector/6 -> [Te], Te/1, Scope5/1  "<Electromagnetic torque Te (N*m)>"
  Gain/1 -> [wm1], 电机轴角速度/1  "转每分钟"
  Clark/1(Alpha) -> Park/1(Alpha), [alpha_k]
  Clark/2(Beta) -> Park/2(Beta), [beta_k]
  [Ia] -> Clark/1(A)
  [Ib] -> Clark/2(B)
  [Ic] -> Clark/3(C)
  极对数/1 -> Park/3(angle), Scope18/1
  Park/1(D) -> [id_k]  "id"
  Park/2(Q) -> [iq_k]  "iq"
  [switch] -> Universal Bridge/1
  Mux1/1 -> Scope/1
  Gain1/1 -> 2_vector_MPC_control1/8(dtheta_e)
  Constant12/1 -> 2_vector_MPC_control1/6(Ld)
  Constant11/1 -> 2_vector_MPC_control1/7(Lq)
  Constant13/1 -> 2_vector_MPC_control1/5(flux)
  [Teref] -> Rate Transition5/1
  [phi_s_ref] -> Rate Transition6/1
  [iq_k] -> Rate Transition/1
  [id_k] -> Rate Transition1/1
  [theta] -> Rate Transition2/1
  [wm] -> Rate Transition3/1
  [Te] -> Rate Transition4/1
  参考转矩/1 -> Add/1
  补偿转矩/1 -> Add/2
  Add/1 -> [Teref]
  connections:
  Universal Bridge/LConn2 -- Permanent Magnet Synchronous Machine1/LConn2
  Universal Bridge/LConn3 -- Permanent Magnet Synchronous Machine1/LConn3
  Universal Bridge/LConn1 -- Permanent Magnet Synchronous Machine1/LConn1
  DC/RConn1 -- Universal Bridge/RConn1
  DC/LConn1 -- Universal Bridge/RConn2

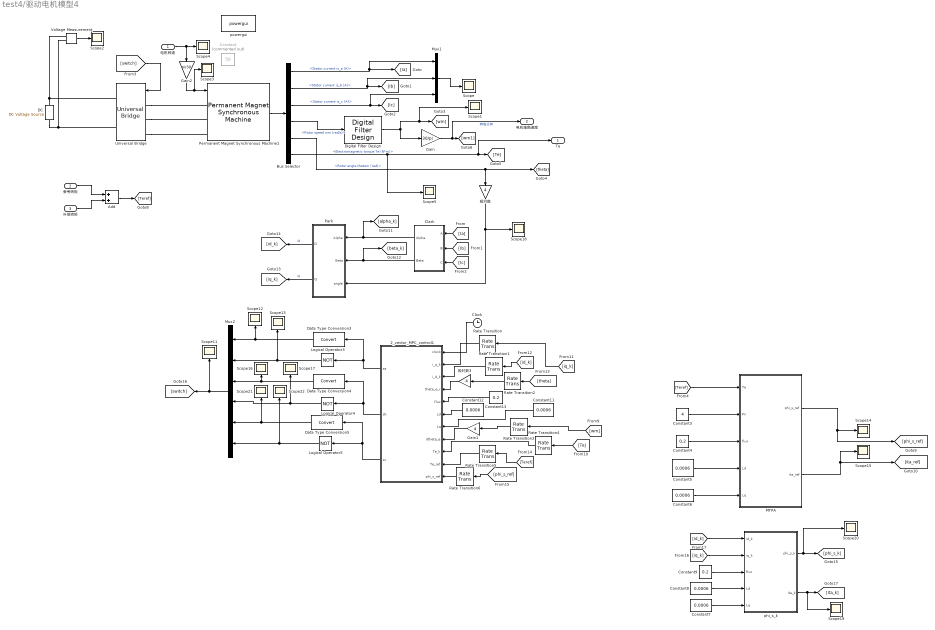
== system test4/驱动电机模型4 ==
  电机转速 : Inport
  参考转矩 : Inport  Port=2
  补偿转矩 : Inport  Port=3
  2_vector_MPC_control1 : MATLAB Function  TreatAsAtomicUnit=on  SystemSampleTime=1e-5
  Add : Sum
  Bus Selector : BusSelector  OutputSignals=Stator current is_a (A),Stator current is_b (A),Stator current is_c (A),Rotor speed wm (rad/s),Rotor angle thetam (rad),Electromagnetic torque Te (N*m)
  Clark : Subsystem
  Clock : Clock
  Constant : Constant  Commented=on  Value=50
  Constant{5..8,11..12} (6 alike) : Constant  Value=0.0006
  Constant13 : Constant  Value=0.2
  Constant3 : Constant  Value=4
  Constant4 : Constant  Value=0.2
  Constant9 : Constant  Value=0.2
  DC : spsDCVoltageSourceLib/DC Voltage Source  Amplitude=400  Measurements=None
  Data Type Conversion3 : DataTypeConversion
  Data Type Conversion4 : DataTypeConversion
  Data Type Conversion5 : DataTypeConversion
  Digital Filter Design : dsparch4/Digital Filter Design  mwdsp_browser_bugfix_var=off
  Gain : Gain  Gain=30/pi
  Gain1 : Gain  Gain=4
  Gain2 : Gain  Gain=pi/30
  Logical Operator3 : Logic  Operator=NOT  AllPortsSameDT=off  OutDataTypeStr=boolean
  Logical Operator4 : Logic  Operator=NOT  AllPortsSameDT=off  OutDataTypeStr=boolean
  Logical Operator5 : Logic  Operator=NOT  AllPortsSameDT=off  OutDataTypeStr=boolean
  MTPA : MATLAB Function  TreatAsAtomicUnit=on
  Mux1 : Mux  Inputs=3
  Mux2 : Mux  Inputs=6
  Park : Subsystem
  Permanent Magnet Synchronous Machine1 : spsPermanentMagnetSynchronousMachineLib/Permanent Magnet Synchronous Machine  NbPhases=3  FluxDistribution=Sinusoidal  RotorType=Salient-pole  MechanicalLoad=Speed w  PresetModel=No  ShowDetailedParameters=on  MeasurementBus=off  Resistance=0.01  Inductance=8.5e-3  dqInductances=[0.0006 0.0006]  La=0.000835  MachineConstant=Flux linkage established by magnets (V.s)  Flux=0.2  VoltageCst=145.1039  TorqueCst=1.2  Flat=120  Mechanical=[0.04 0.0002024 4 0]  PolePairs=4  InitialConditions=[0,0, 0,0]  InitialConditions5ph=[0 0 0 0 0 0]  RefAngle=Aligned with phase A axis (original Park)  IterativeDiscreteModel=Trapezoidal non iterative  TsBlock=-1  TsPowergui=0
  Rate Transition : RateTransition  OutPortSampleTime=1e-5
  Rate Transition1 : RateTransition  OutPortSampleTime=1e-5
  Rate Transition2 : RateTransition  OutPortSampleTime=1e-5
  Rate Transition{3..6} (4 alike) : RateTransition  OutPortSampleTime=1e-4
  Scope{,1..5,11..22} (18 alike) : Scope
  Universal Bridge : spsUniversalBridgeLib/Universal Bridge  Arms=3  SnubberResistance=1e5  SnubberCapacitance=inf  Device=IGBT / Diodes  Ron=1e-3  Lon=0  ForwardVoltages="[  0  0  ]"  ForwardVoltage=0  GTOparameters=[ 10e-6 , 20e-6 ]  IGBTparameters=[ 1e-6 , 2e-6 ]  Measurements=None  Measurements_2=None  converterType=Rectifier
  Voltage Measurement : spsVoltageMeasurementLib/Voltage Measurement  PhasorSimulation=off  OutputType=Complex  PSBequivalent=0
  phi_s_k : MATLAB Function  TreatAsAtomicUnit=on
  powergui : spspowerguiLib/powergui  Priority=1  SimulationMode=Discrete  SampleTime=1e-6  frequency=60  Iterations=50  frequencyindice=0  Pbase=100e6  ErrMax=1e-4  UnitsV=kV  UnitsW=MW  buscounter=0  FunctionMessages=off  echomessages=off  EnableUseOfTLC=off  CurrentSourceSwitches=off  DisableSnubberDevices=off  DisableRonSwitches=off  DisableVfSwitches=off  DisplayEquations=off  AutomaticDiscreteSolvers=off  SolverType=Tustin/Backward Euler (TBE)  Interpol=off  ExternalGateDelay=off  methode=off  Ts=100  x0status=blocks  SPID=on  SwTol=0  HookPort=off  NonlinearTolerance=1e-4  nMaxIteration=100  ContinueOnMaxIteration=off  RestoreLinks=warning  ResistiveCurrentMeasurement=off  Frange=[0:2:500]  Ylog=off  Xlog=on  ShowGrid=off  save=off  variable=ZData  structure=0  ZoomFFT=off  StartTime=0.0  cycles=1  DisplayStyle=1  fundamental=60  FreqAxis=off  MaxFrequency=1000  frequencyindicesteady=1  RmsSteady=1  display=off
  极对数 : Gain  Gain=4
  极对数3 : Gain  Gain=4
  Te : Outport
  电机轴角速度 : Outport  Port=2
  wires:
  Constant13/1 -> 2_vector_MPC_control1/5(flux)
  Digital Filter Design/1 -> Gain/1, Scope1/1, [wm]
  Gain2/1 -> Permanent Magnet Synchronous Machine1/1, Scope3/1
  电机转速/1 -> Gain2/1, Scope4/1
  Rate Transition6/1 -> 2_vector_MPC_control1/11(phi_s_ref)
  Rate Transition5/1 -> 2_vector_MPC_control1/10(Te_ref)
  Rate Transition4/1 -> 2_vector_MPC_control1/9(Te_k)
  Rate Transition3/1 -> Gain1/1
  Rate Transition2/1 -> 极对数3/1
  Rate Transition1/1 -> 2_vector_MPC_control1/3(i_d_k)
  Rate Transition/1 -> 2_vector_MPC_control1/2(i_q_k)
  phi_s_k/2(ita_k) -> [ita_k], Scope19/1
  极对数3/1 -> 2_vector_MPC_control1/4(theta_e_r)
  Mux2/1 -> [switch], Scope11/1
  Logical Operator5/1 -> Scope22/1, Mux2/6
  Data Type Conversion5/1 -> Scope21/1, Mux2/5
  Logical Operator4/1 -> Scope17/1, Mux2/4
  Data Type Conversion4/1 -> Scope16/1, Mux2/3
  Logical Operator3/1 -> Scope13/1, Mux2/2
  Data Type Conversion3/1 -> Scope12/1, Mux2/1
  2_vector_MPC_control1/3(sc) -> Logical Operator5/1, Data Type Conversion5/1
  2_vector_MPC_control1/2(sb) -> Logical Operator4/1, Data Type Conversion4/1
  2_vector_MPC_control1/1(sa) -> Logical Operator3/1, Data Type Conversion3/1
  [id_k] -> phi_s_k/1(id_k)
  [iq_k] -> phi_s_k/2(iq_k)
  phi_s_k/1(phi_s_k) -> Scope20/1, [phi_s_k]
  Constant9/1 -> phi_s_k/3(flux)
  Constant8/1 -> phi_s_k/4(Ld)
  Constant7/1 -> phi_s_k/5(Lq)
  MTPA/1(phi_s_ref) -> Scope14/1, [phi_s_ref]
  MTPA/2(ita_ref) -> [ita_ref], Scope15/1
  Constant6/1 -> MTPA/5(Lq)
  Constant5/1 -> MTPA/4(Ld)
  Constant4/1 -> MTPA/3(flux)
  Constant3/1 -> MTPA/2(Pn)
  [Teref] -> MTPA/1(Te)
  Clock/1 -> 2_vector_MPC_control1/1(clock)
  Permanent Magnet Synchronous Machine1/1 -> Bus Selector/1
  Bus Selector/1 -> Mux1/1, [Ia]  "<Stator current is_a (A)>"
  Bus Selector/2 -> Mux1/2, [Ib]  "<Stator current is_b (A)>"
  Bus Selector/3 -> Mux1/3, [Ic]  "<Stator current is_c (A)>"
  Bus Selector/4 -> Digital Filter Design/1  "<Rotor speed wm (rad/s)>"
  Bus Selector/5 -> 极对数/1, [theta]  "<Rotor angle thetam (rad)>"
  Bus Selector/6 -> [Te], Te/1, Scope5/1  "<Electromagnetic torque Te (N*m)>"
  Gain/1 -> [wm1], 电机轴角速度/1  "转每分钟"
  Clark/1(Alpha) -> Park/1(Alpha), [alpha_k]
  Clark/2(Beta) -> [beta_k], Park/2(Beta)
  [Ia] -> Clark/1(A)
  [Ib] -> Clark/2(B)
  [Ic] -> Clark/3(C)
  极对数/1 -> Park/3(angle), Scope18/1
  Park/1(D) -> [id_k]  "id"
  Park/2(Q) -> [iq_k]  "iq"
  [switch] -> Universal Bridge/1
  Mux1/1 -> Scope/1
  Gain1/1 -> 2_vector_MPC_control1/8(dtheta_e)
  Constant12/1 -> 2_vector_MPC_control1/6(Ld)
  Constant11/1 -> 2_vector_MPC_control1/7(Lq)
  [Teref] -> Rate Transition5/1
  [phi_s_ref] -> Rate Transition6/1
  [iq_k] -> Rate Transition/1
  [id_k] -> Rate Transition1/1
  [theta] -> Rate Transition2/1
  [wm] -> Rate Transition3/1
  [Te] -> Rate Transition4/1
  补偿转矩/1 -> Add/2
  Add/1 -> [Teref]
  参考转矩/1 -> Add/1
  Voltage Measurement/1 -> Scope2/1
  connections:
  Universal Bridge/LConn2 -- Permanent Magnet Synchronous Machine1/LConn2
  Universal Bridge/LConn3 -- Permanent Magnet Synchronous Machine1/LConn3
  DC/RConn1 -- Voltage Measurement/LConn1 -- Universal Bridge/RConn1
  DC/LConn1 -- Voltage Measurement/LConn2 -- Universal Bridge/RConn2
  Universal Bridge/LConn1 -- Permanent Magnet Synchronous Machine1/LConn1

== system test4/驾驶员模型1 ==
  参考转速 : Inport
  电机转速 : Inport  Port=2
  Add : Sum  Inputs=+++
  Constant : Constant  Value=0
  Constant2 : Constant  Value=0
  Constant3 : Constant
  Constant4 : Constant  Value=2
  Gain : Gain  Gain=1/200
  PID Controller : pid_lib/PID Controller  Controller=PID  Form=Parallel  TimeDomain=Continuous-time  UseExternalTs=off  SampleTime=-1  IntegratorMethod=Forward Euler  FilterMethod=Forward Euler  ControllerParametersSource=internal  P=2  I=0.125  D=0.01  UseFilter=on  N=100  TunerSelectOption=Transfer Function Based (PID Tuner App)  InitialConditionSource=internal  InitialConditionForIntegrator=0  InitialConditionForFilter=0  DifferentiatorICPrevScaledInput=0  ExternalReset=none  TrackingMode=off  Kt=1  LimitOutput=on  SatLimitsSource=internal  UpperSaturationLimit=200  LowerSaturationLimit=-200  LinearizeAsGain=on  AntiWindupMode=none  Kb=1  POutMin=[]  POutMax=[]  IOutMin=[]  IOutMax=[]  DOutMin=[]  DOutMax=[]  NOutMin=[]  NOutMax=[]  SumOutMin=[]  SumOutMax=[]  SaturationOutMin=[]  SaturationOutMax=[]  PParamMin=[]  PParamMax=[]  IParamMin=[]  IParamMax=[]  DParamMin=[]  DParamMax=[]  NParamMin=[]  NParamMax=[]  KbParamMin=[]  KbParamMax=[]  KtParamMin=[]  KtParamMax=[]  KbOutMin=[]  KbOutMax=[]  KtOutMin=[]  KtOutMax=[]  IntegratorOutMin=[]  IntegratorOutMax=[]  FilterOutMin=[]  FilterOutMax=[]  SumI1OutMin=[]  SumI1OutMax=[]  SumI2OutMin=[]  SumI2OutMax=[]  SumI3OutMin=[]  SumI3OutMax=[]  SumI4OutMin=[]  SumI4OutMax=[]  SumDOutMin=[]  SumDOutMax=[]  DifferentiatorOutMin=[]  DifferentiatorOutMax=[]  FilterDiffOutCoefMin=[]  FilterDiffOutCoefMax=[]  ReciprocalOutMin=[]  ReciprocalOutMax=[]  SumDenOutMin=[]  SumDenOutMax=[]  SumNumOutMin=[]  SumNumOutMax=[]  DivideOutMin=[]  DivideOutMax=[]  UdiffTsProdOutMin=[]  UdiffTsProdOutMax=[]  NTsProdOutMin=[]  NTsProdOutMax=[]  UintegralTsProdOutMin=[]  UintegralTsProdOutMax=[]  UngainTsProdOutMin=[]  UngainTsProdOutMax=[]  IntegratorContinuousStateAttributes=''  IntegratorStateMustResolveToSignalObject=off  IntegratorRTWStateStorageClass=Auto  FilterContinuousStateAttributes=''  FilterStateMustResolveToSignalObject=off  FilterRTWStateStorageClass=Auto  ParallelPVariant=InternalParameters  IdealPVariant=Disabled  IVariant=InternalParameters  DVariant=InternalParameters  IntegratorVariant=Continuous  SatVariant=Enabled  AWVariant=Passthrough  PCopyVariant=Disabled  TRVariant=Disabled  FdbkBlocksVariant=Forward  IdealPFdbkVariant=Disabled  SatFdbkVariant=Disabled  DerivativeFilterVariant=ContFilter  NVariant=InternalParameters  NCopyVariant=Disabled  FilterICVariant=InternalICsFilter  IntegratorICVariant=InternalICs  ExternalResetVariant=Disabled  TRSumVariant=Passthrough  SumFdbkVariant=Disabled  SumVariant=Sum_PID  TsampFilterVariant=InternalTs  TsampNgainVariant=Passthrough  TsampIntegralVariant=Passthrough  ExternalSaturationOutDataTypeStr=Inherit: Same as second input
  Relational Operator : RelationalOperator  Operator=>  OutDataTypeStr=boolean  RndMeth=Simplest
  Relational Operator1 : RelationalOperator  Operator=<  OutDataTypeStr=boolean  RndMeth=Simplest
  Scope1 : Scope
  Scope10 : Scope
  Scope11 : Scope
  Sum : Sum  Inputs=|+-
  Switch : Switch  Threshold=1
  Switch1 : Switch  Threshold=1
  Switch2 : Switch  Criteria=u2 ~= 0  Threshold=1
  参考转矩 : Outport
  电机驱动/制动模式 : Outport  Port=2
  wires:
  Constant/1 -> Switch2/3
  PID Controller/1 -> Switch2/1
  Switch2/1 -> Gain/1, 参考转矩/1, Scope10/1
  参考转速/1 -> Sum/1, Switch2/2
  Add/1 -> 电机驱动/制动模式/1, Scope1/1
  Switch1/1 -> Add/2
  Switch/1 -> Add/1
  Constant4/1 -> Switch1/1
  Relational Operator1/1 -> Switch1/2
  Constant3/1 -> Switch/1
  Relational Operator/1 -> Switch/2
  Constant2/1 -> Relational Operator/2, Switch/3, Relational Operator1/2, Switch1/3, Add/3
  Gain/1 -> Relational Operator/1, Relational Operator1/1  "期望加速度强度"
  Sum/1 -> PID Controller/1
  电机转速/1 -> Sum/2, Scope11/1
